simulink model "Motor_citizen_PWM_simu"  (Simulink 7.1)
settings: Solver=ode15s  StartTime=0.0  StopTime=1  RelTol=1e-3
libraries: fl_lib x13, simulink x4, nesl_utility x4
settings Model: Creator=cell  LastModifiedBy=cell
settings DebuggingCC: SolverPrmCheckMsg=none

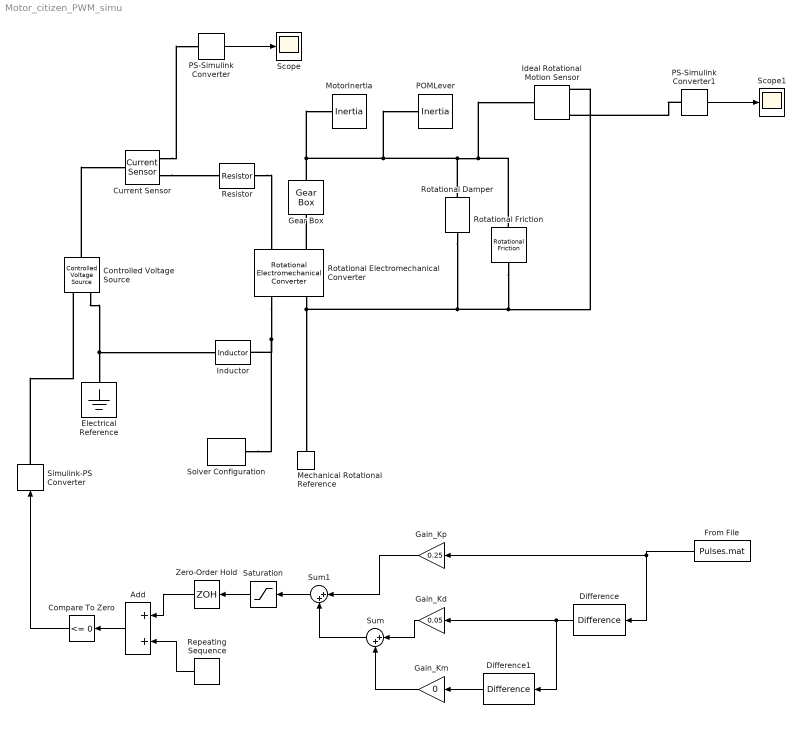
== system Motor_citizen_PWM_simu ==
  Add : Sum  Orientation=left  OutDataType=sfix(16)  OutScaling=2^-10
  Compare To Zero : simulink/Logic and Bit Operations/Compare To Zero  Orientation=left  SystemSampleTime=-1  relop=<=  LogicOutDataTypeMode=uint8  ZeroCross=off
  Controlled Voltage Source : fl_lib/Electrical/Electrical Sources/Controlled Voltage Source  Orientation=down  DialogController=NetworkEngine.DynNeDlgSource  SystemSampleTime=-1  current_Log=off  voltage_Log=off  power_Log=off  LocalVarNames=|current|voltage|power  LocalVarDescs=|Current (A)|Voltage (V)|Power (W)  LocalVarLogging=[0 0 0]
  Current Sensor : fl_lib/Electrical/Electrical Sensors/Current Sensor  DialogController=NetworkEngine.DynNeDlgSource  SystemSampleTime=-1  LocalVarLogging=[]
  Difference : simulink/Discrete/Difference  Orientation=left  SystemSampleTime=-1  ICPrevInput=0.0  OutMin=[]  OutMax=[]  OutDataType=sfix(16)  OutScaling=2^-10  DoSatur=off
  Difference1 : simulink/Discrete/Difference  Orientation=left  SystemSampleTime=-1  ICPrevInput=0.0  OutMin=[]  OutMax=[]  OutDataType=sfix(16)  OutScaling=2^-10  DoSatur=off
  Electrical Reference : fl_lib/Electrical/Electrical Elements/Electrical Reference  Orientation=down  DialogController=NetworkEngine.DynNeDlgSource  SystemSampleTime=-1  LocalVarLogging=[]
  From File : FromFile  Orientation=left  FileName=Pulses.mat  SampleTime=0.001
  Gain_Kd : Gain  Orientation=left  Gain=0.05  ParameterDataType=sfix(16)  ParameterScaling=2^0  OutDataType=sfix(16)  OutScaling=2^0
  Gain_Km : Gain  Orientation=left  Gain=0  ParameterDataType=sfix(16)  ParameterScaling=2^0  OutDataType=sfix(16)  OutScaling=2^0
  Gain_Kp : Gain  Orientation=left  Gain=0.25  ParameterDataType=sfix(16)  ParameterScaling=2^0  OutDataType=sfix(16)  OutScaling=2^0
  Gear Box : fl_lib/Mechanical/Mechanisms/Gear Box  Orientation=up  DialogController=NetworkEngine.DynNeDlgSource  SystemSampleTime=-1  ratio=15.58  torque_inp_Log=off  ang_velocity_inp_Log=off  power_Log=off  LocalVarNames=|torque_inp|ang_velocity_inp|power  LocalVarDescs=|Input shaft torque (N*m)|Input shaft angular velocity (rad/s)|Power transmitted by the box (W)  LocalVarLogging=[0 0 0]
  Ideal Rotational Motion Sensor : fl_lib/Mechanical/Mechanical Sensors and Sources/Ideal Rotational Motion Sensor  DialogController=NetworkEngine.DynNeDlgSource  SystemSampleTime=-1  offset=0 rad  LocalVarLogging=[]
  Inductor : fl_lib/Electrical/Electrical Elements/Inductor  DialogController=NetworkEngine.DynNeDlgSource  SystemSampleTime=-1  l=464e-06 H  i0=0 A  r=0 Ohm  g=1e-09 1/Ohm  current_Log=off  voltage_Log=off  power_Log=off  LocalVarNames=|current|voltage|power  LocalVarDescs=|Inductor current (A) |Voltage across inductor (V)|Power (W)  LocalVarLogging=[0 0 0]
  Mechanical Rotational Reference : fl_lib/Mechanical/Rotational Elements/Mechanical Rotational Reference  Orientation=down  DialogController=NetworkEngine.DynNeDlgSource  SystemSampleTime=-1  LocalVarLogging=[]
  MotorInertia : fl_lib/Mechanical/Rotational Elements/Inertia  DialogController=NetworkEngine.DynNeDlgSource  SystemSampleTime=-1  inertia=0.841 g*cm^2  initial_velocity=0 rad/s  torque_Log=off  velocity_Log=off  LocalVarNames=|torque|velocity  LocalVarDescs=|Inertia torque (N*m)|Inertia absolute velocity (rad/s)  LocalVarLogging=[0 0]
  POMLever : fl_lib/Mechanical/Rotational Elements/Inertia  DialogController=NetworkEngine.DynNeDlgSource  SystemSampleTime=-1  inertia=1.613 g*cm^2  initial_velocity=0 rad/s  torque_Log=off  velocity_Log=off  LocalVarNames=|torque|velocity  LocalVarDescs=|Inertia torque (N*m)|Inertia absolute velocity (rad/s)  LocalVarLogging=[0 0]
  PS-Simulink Converter : nesl_utility/PS-Simulink Converter  DialogController=NetworkEngine.DynNeUtilDlgSource  SystemSampleTime=-1  PhysicalDomain=network_engine_domain  LeftPortType=input  RightPortType=output  SubClassName=ps_output  Unit=A  AffineConversion=off
  PS-Simulink Converter1 : nesl_utility/PS-Simulink Converter  DialogController=NetworkEngine.DynNeUtilDlgSource  SystemSampleTime=-1  PhysicalDomain=network_engine_domain  LeftPortType=input  RightPortType=output  SubClassName=ps_output  Unit=deg  AffineConversion=off
  Repeating Sequence : simulink/Sources/Repeating Sequence  Orientation=left  SystemSampleTime=-1  rep_seq_t=[0 0.00005]  rep_seq_y=[-1 1]
  Resistor : fl_lib/Electrical/Electrical Elements/Resistor  DialogController=NetworkEngine.DynNeDlgSource  SystemSampleTime=-1  R=14 Ohm  current_Log=off  voltage_Log=off  power_Log=off  LocalVarNames=|current|voltage|power  LocalVarDescs=|Resistor current (A)|Voltage across resistor (V)|Power (W)  LocalVarLogging=[0 0 0]
  Rotational Electromechanical Converter : fl_lib/Electrical/Electrical Elements/Rotational Electromechanical Converter  Orientation=down  DialogController=NetworkEngine.DynNeDlgSource  SystemSampleTime=-1  K=0.01807 V/(rad/s)  current_Log=off  voltage_Log=off  power_Log=off  torque_Log=off  speed_Log=off  LocalVarNames=|current|voltage|power|torque|speed  LocalVarDescs=|Current (A)|Voltage (V)|Power (W)|Torque (Nm)|Angular speed (rad/s)  LocalVarLogging=[0 0 0 0 0]
  Rotational Damper : fl_lib/Mechanical/Rotational Elements/Rotational Damper  Orientation=down  DialogController=NetworkEngine.DynNeDlgSource  SystemSampleTime=-1  D=0.001 N*m/(rad/s)  torque_Log=off  velocity_Log=off  power_Log=off  LocalVarNames=|torque|velocity|power  LocalVarDescs=|Damping torque (N*m)|Damper relative velocity (rad/s)|Power dissipated in the damper (W)  LocalVarLogging=[0 0 0]
  Rotational Friction : fl_lib/Mechanical/Rotational Elements/Rotational Friction  Orientation=down  DialogController=NetworkEngine.DynNeDlgSource  SystemSampleTime=-1  brkwy_trq=0.02e-3 N*m  Col_trq=0.02e-3 N*m  visc_coef=0.0 N*m/(rad/s)  trans_coef=10 s/rad  vel_thr=0.1 rad/s  friction_torque_Log=off  rel_velocity_Log=off  power_Log=off  LocalVarNames=|friction_torque|rel_velocity|power  LocalVarDescs=|Friction torque (N*m)|Relative velocity (rad/s)|Power (W)  LocalVarLogging=[0 0 0]
  Saturation : Saturate  Orientation=left  UpperLimit=0.9  LowerLimit=-0.9  OutDataType=sfix(16)  OutScaling=2^0
  Scope : Scope
  Scope1 : Scope
  Simulink-PS Converter : nesl_utility/Simulink-PS Converter  Orientation=up  DialogController=NetworkEngine.DynNeUtilDlgSource  SystemSampleTime=-1  PhysicalDomain=network_engine_domain  LeftPortType=input  RightPortType=output  SubClassName=ps_input  Unit=V  AffineConversion=off
  Solver Configuration : nesl_utility/Solver Configuration  DialogController=NetworkEngine.DynNeUtilDlgSource  SystemSampleTime=-1  PhysicalDomain=network_engine_domain  LeftPortType=input  RightPortType=generic  SubClassName=solver  Accelerate=off  Profile=off  ResidualTolerance=1e-9  MaxNonlinIter=12  MaxModeIter=2  DoFixedCost=off  DoDC=off  LinearAlgebra=Sparse
  Sum : Sum  Orientation=left  Inputs=|++  OutDataType=sfix(16)  OutScaling=2^0
  Sum1 : Sum  Orientation=left  Inputs=|++  OutDataType=sfix(16)  OutScaling=2^0
  Zero-Order Hold : ZeroOrderHold  Orientation=left
  wires:
  PS-Simulink Converter/1 -> Scope/1
  PS-Simulink Converter1/1 -> Scope1/1
  From File/1 -> Gain_Kp/1, Difference/1
  Difference/1 -> Gain_Kd/1, Difference1/1
  Difference1/1 -> Gain_Km/1
  Gain_Kd/1 -> Sum/1
  Gain_Km/1 -> Sum/2
  Gain_Kp/1 -> Sum1/1
  Sum/1 -> Sum1/2
  Sum1/1 -> Saturation/1
  Saturation/1 -> Zero-Order Hold/1
  Compare To Zero/1 -> Simulink-PS Converter/1
  Zero-Order Hold/1 -> Add/1
  Repeating Sequence/1 -> Add/2
  Add/1 -> Compare To Zero/1
  connections:
  Controlled Voltage Source/LConn1 -- Current Sensor/LConn1
  Current Sensor/RConn2 -- Resistor/LConn1
  Controlled Voltage Source/RConn2 -- Inductor/LConn1 -- Electrical Reference/LConn1
  Current Sensor/RConn1 -- PS-Simulink Converter/LConn1
  Resistor/RConn1 -- Rotational Electromechanical Converter/LConn1
  Rotational Electromechanical Converter/RConn1 -- Inductor/RConn1 -- Solver Configuration/RConn1
  Ideal Rotational Motion Sensor/RConn1 -- Rotational Electromechanical Converter/RConn2 -- Mechanical Rotational Reference/LConn1 -- Rotational Damper/RConn1 -- Rotational Friction/RConn1
  Ideal Rotational Motion Sensor/LConn1 -- Rotational Friction/LConn1 -- Rotational Damper/LConn1 -- MotorInertia/LConn1 -- Gear Box/RConn1 -- POMLever/LConn1
  PS-Simulink Converter1/LConn1 -- Ideal Rotational Motion Sensor/RConn3
  Rotational Electromechanical Converter/LConn2 -- Gear Box/LConn1
  Simulink-PS Converter/RConn1 -- Controlled Voltage Source/RConn1
